simulink model "GOcontroll_Linux"  (R2018b)
settings: Solver=FixedStepDiscrete  StartTime=0.0  StopTime=5  FixedStep=0.01  RelTol=1e-3
PreLoadFcn:
  | librarySetup
PostLoadFcn:
  | core_info = evalc('feature(''numcores'')');
  | core_info_split = split(core_info, " ");
  | num_cores = core_info_split{12};
  | set_param(bdroot, "MakeCommand", ['make_rtw -j' num_cores]);
  | clear num_cores core_info core_info_split
libraries: GOcontroll_Moduline_Target x35, GOcontroll_Modbus x21, simulink x13, hdlsllib x8
settings Model: Creator=la_obwlf  LastModifiedBy=maud
settings DataIOCC: LimitDataPoints=on  SaveFormat=Array
settings OptimizationCC: BlockReduction=off  DefaultParameterBehavior=Inlined  LifeSpan=1
settings DebuggingCC: SolverPrmCheckMsg=warning  MultiTaskRateTransMsg=warning  ParameterPrecisionLossMsg=none  UnconnectedLineMsg=none  SFUnusedDataAndEventsDiag=none  SFUnexpectedBacktrackingDiag=warning  SFNoUnconditionalDefaultTransitionDiag=warning  SFUndirectedBroadcastEventsDiag=none  SFExecutionAtInitializationDiag=none  RCSCRenamedMsg=none  RCSCObservableMsg=none
settings HardwareCC: ProdBitPerLong=64  ProdLargestAtomicInteger=Long  ProdLargestAtomicFloat=Double  ProdLongLongMode=on  ProdHWDeviceType=ARM Compatible->ARM 64-bit (LP64)
settings ModelReferenceCC: PropagateSignalLabelsOutOfModel=off
settings SFSimCC: SimUseLocalCustomCode=off  MATLABDynamicMemAlloc=off
settings RTWCC: SystemTargetFile=ert_linux.tlc  MakeCommand=make_rtw -j24  TemplateMakefile=ert_linux_target_64.tmf  Description=Linux Embedded Coder  RTWUseLocalCustomCode=off
settings CodeAppCC: IgnoreCustomStorageClasses=off  StateflowObjectComments=on
settings STFCustomTargetCC: CombineOutputUpdateFcns=on  ERTCustomFileBanners=on  SupportContinuousTime=off  SupportNonInlinedSFcns=off  RemoveResetFunc=on  MATLABClassNameForMDSCustomization=Simulink.SoftwareTarget.ERTCustomization  SystemTargetFile=ert_linux.tlc
settings ERTTargetCC: MultiwordLength=2048  ParMdlRefBuildCompliant=off  CompOptLevelCompliant=off  ConcurrentExecutionCompliant=off  ModelStepFunctionPrototypeControlCompliant=off  CPPClassGenCompliant=off  UseToolchainInfoCompliant=off  GenerateASAP2=on  ERTCustomFileTemplate=ert_linux_file_process.tlc  PreserveExpressionOrder=on  ConvertIfToSwitch=off  SuppressUnreachableDefaultCases=off
settings ConfigComp: CovMetricSettings=dw  CovHtmlReporting=on  CovSaveCumulativeToWorkspaceVar=on  CovSaveSingleToWorkspaceVar=on  CovExternalEMLEnable=off  CovSFcnEnable=off

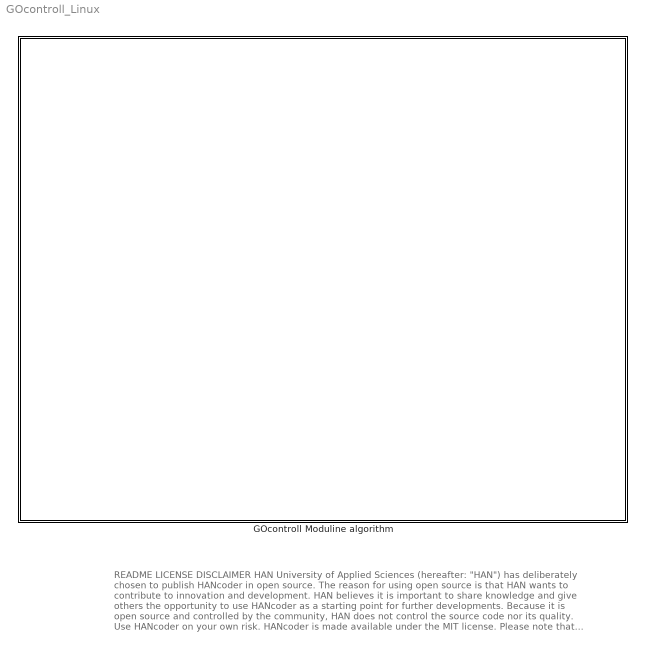
== system GOcontroll_Linux ==
  note: README
      |
      | LICENSE
      |
      | DISCLAIMER
      |
      | HAN University of Applied Sciences (hereafter: "HAN") has deliberately chosen
      | to publish HANcoder in open source. The reason for using open source is that
      | HAN wants to contribute to innovation and development. HAN believes it is
      | important to share knowledge and give others the opportunity to use HANcoder
      | as a starting point for further developments. Because it is open source and
      | controlled by the community, HAN does not control the source code nor its
      | quality. Use HANcoder on your own risk. HANcoder is made available under the
      | MIT license. Please note that this license contains an exclusion of liability.
  GOcontroll Moduline algorithm : Subsystem  mask(TopLevelSubsystem){}
      mask Display: image(imread('GOcontroll.png'))

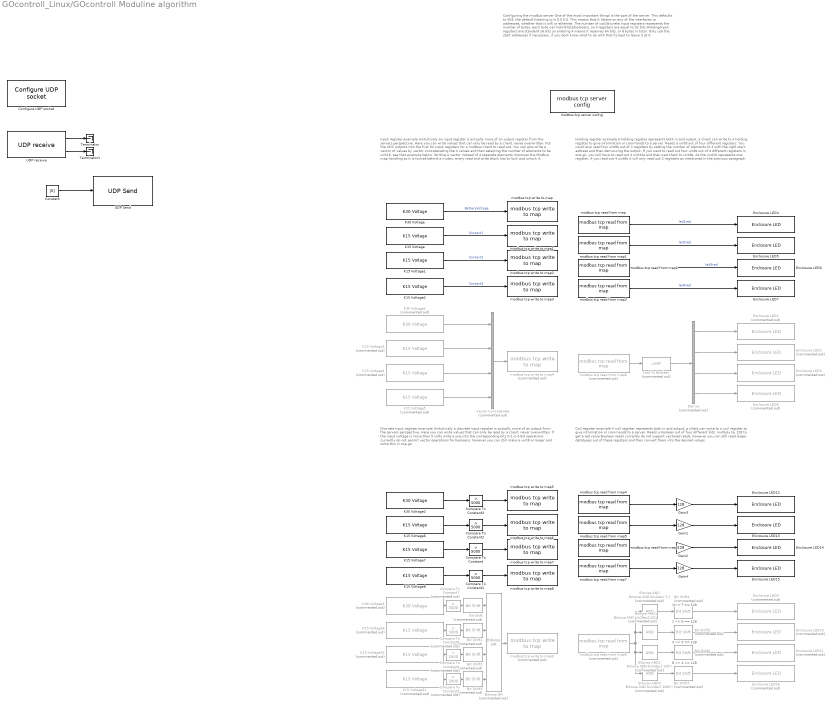
== system GOcontroll_Linux/GOcontroll Moduline algorithm ==
  note: 1 << 7 == 128
  note: Configuring the modbus server
      | One of the most important things is the port of the server.
      | This defaults to 503, the default listening ip is 0.0.0.0.
      | This means that it listens on any of the interfaces ip addresses,
      | whether that is wifi or ethernet.
      |
      | The number of coil/discrete input registers represents the number of bytes,
      | each byte can hold 8 bits/booleans, so 4 registers are equal to 32 bits
      |
      | Holding/input registers are standard 16 bits so entering 4 means it reserves
      | 64 bits, or 8 bytes in total.
      |
      | Only use the start addresses if necessary, if you dont know what to do with that
      | its best to leave it at 0
  note: Holding register example
      | A holding register represents both in and output, a client can write
      | to a holding register to give information or commands to a server.
      |
      | Reads a uint8 out of four different registers.
      | You could also read four uint8s out of 2 registers by setting
      | the number of elements to 4 with the right start address and then
      | demuxxing the output.
      |
      | If you want to read out four uin8s out of 4 different registers in one go, you will have to read out 4 uint16s
      | and then cast them to uint8s. As the uint16 represents one register, if you read out 4 uint8s it will only read out 2
      | registers as mentioned in the previous paragraph
  note: Input register example
      | Unituitively an input register is actually more of an output register from the servers perspective.
      | Here you can write values that can only be read by a client, never overwritten.
      |
      | Put the ADC outputs into the first for input registers for a modbus client to read out.
      |
      | You can also write a vector of values by vector concatenating the 4 values and then selecting
      | the number of elements to be uint16, see that example below.
      | Writing a vector instead of 4 seperate elements improves the Modbus map handling as it is
      | locked behind a mutex, every read and write block has to lock and unlock it.
  note: Coil register example
      | A coil register represents both in and output, a client can write
      | to a coil register to give information or commands to a server.
      |
      | Reads a boolean out of four different bits, multiply by 128 to get a led value
      |
      | Boolean reads currently do not support vectored reads, however you can still read larger datatypes out of these
      | registers and then convert them into the desired values.
  note: Discrete input register example
      | Unituitively a discrete input register is actually more of an output from the servers perspective.
      | Here you can write values that can only be read by a client, never overwritten.
      |
      | If the input voltage is more than 5 volts write a one into the corresponding bits 0-1-2-3
      |
      | Bit operations currently do not permit vector operations for booleans, however you can still
      | make a uint8 or larger and write this in one go.
  note: 2 << 6 == 128
  note: 4 << 5 == 128
  note: 8 << 4 == 128
  Bit Shift : hdlsllib/Logic and Bit Operations/Bit Shift  Commented=on  mode=Shift Left Logical  N=0
      settings: SourceProductName=HDL Coder  SourceProductBaseCode=HD
  Bit Shift1 : hdlsllib/Logic and Bit Operations/Bit Shift  Commented=on  mode=Shift Left Logical  N=1
      settings: SourceProductName=HDL Coder  SourceProductBaseCode=HD
  Bit Shift2 : hdlsllib/Logic and Bit Operations/Bit Shift  Commented=on  mode=Shift Left Logical  N=2
      settings: SourceProductName=HDL Coder  SourceProductBaseCode=HD
  Bit Shift3 : hdlsllib/Logic and Bit Operations/Bit Shift  Commented=on  mode=Shift Left Logical  N=3
      settings: SourceProductName=HDL Coder  SourceProductBaseCode=HD
  Bit Shift4 : hdlsllib/Logic and Bit Operations/Bit Shift  Commented=on  mode=Shift Left Logical  N=7
      settings: SourceProductName=HDL Coder  SourceProductBaseCode=HD
  Bit Shift5 : hdlsllib/Logic and Bit Operations/Bit Shift  Commented=on  mode=Shift Left Logical  N=6
      settings: SourceProductName=HDL Coder  SourceProductBaseCode=HD
  Bit Shift6 : hdlsllib/Logic and Bit Operations/Bit Shift  Commented=on  mode=Shift Left Logical  N=5
      settings: SourceProductName=HDL Coder  SourceProductBaseCode=HD
  Bit Shift7 : hdlsllib/Logic and Bit Operations/Bit Shift  Commented=on  mode=Shift Left Logical  N=4
      settings: SourceProductName=HDL Coder  SourceProductBaseCode=HD
  Bitwise AND : simulink/Logic and Bit Operations/Bitwise Operator  Commented=on  logicop=AND  UseBitMask=on  BitMask=bin2dec('1')  BitMaskRealWorld=Stored Integer
  Bitwise AND1 : simulink/Logic and Bit Operations/Bitwise Operator  Commented=on  logicop=AND  UseBitMask=on  BitMask=bin2dec('10')  BitMaskRealWorld=Stored Integer
  Bitwise AND2 : simulink/Logic and Bit Operations/Bitwise Operator  Commented=on  logicop=AND  UseBitMask=on  BitMask=bin2dec('100')  BitMaskRealWorld=Stored Integer
  Bitwise AND3 : simulink/Logic and Bit Operations/Bitwise Operator  Commented=on  logicop=AND  UseBitMask=on  BitMask=bin2dec('1000')  BitMaskRealWorld=Stored Integer
  Bitwise OR : simulink/Logic and Bit Operations/Bitwise Operator  Commented=on  logicop=OR  UseBitMask=off  NumInputPorts=4  BitMask=bin2dec('11011001')  BitMaskRealWorld=Stored Integer
  Cast To Boolean : DataTypeConversion  Commented=on  OutDataTypeStr=uint8
  Compare To Constant{,1..3} (4 alike) : simulink/Logic and Bit Operations/Compare To Constant  relop=>  const=5000  OutDataTypeStr=boolean
  Compare To Constant{4..7} (4 alike) : simulink/Logic and Bit Operations/Compare To Constant  Commented=on  relop=>  const=5000  OutDataTypeStr=uint8
  Configure UDP socket : GOcontroll_Moduline_Target/Network/UDP/Configure UDP socket  port=9001  ip='0.0.0.0'  broadcast=on  tsamp=0.01
      settings: SourceProductName=GOcontroll Moduline
  Constant : Constant  Value=[0]  OutDataTypeStr=uint8
  Demux : Demux  Commented=on
  Enclosure LED1 : GOcontroll_Moduline_Target/Enclosure LED's/Enclosure LED  Tag=HANcoder_GOcontroll_Moduline_IV  Commented=on  led=1  color=Red
      settings: SourceProductName=GOcontroll Moduline
  Enclosure LED10 : GOcontroll_Moduline_Target/Enclosure LED's/Enclosure LED  Tag=HANcoder_GOcontroll_Moduline_IV  Commented=on  led=2  color=Red
      settings: SourceProductName=GOcontroll Moduline
  Enclosure LED11 : GOcontroll_Moduline_Target/Enclosure LED's/Enclosure LED  Tag=HANcoder_GOcontroll_Moduline_IV  Commented=on  led=3  color=Red
      settings: SourceProductName=GOcontroll Moduline
  Enclosure LED12 : GOcontroll_Moduline_Target/Enclosure LED's/Enclosure LED  Tag=HANcoder_GOcontroll_Moduline_IV  led=1  color=Green
      settings: SourceProductName=GOcontroll Moduline
  Enclosure LED13 : GOcontroll_Moduline_Target/Enclosure LED's/Enclosure LED  Tag=HANcoder_GOcontroll_Moduline_IV  led=2  color=Green
      settings: SourceProductName=GOcontroll Moduline
  Enclosure LED14 : GOcontroll_Moduline_Target/Enclosure LED's/Enclosure LED  Tag=HANcoder_GOcontroll_Moduline_IV  led=3  color=Green
      settings: SourceProductName=GOcontroll Moduline
  Enclosure LED15 : GOcontroll_Moduline_Target/Enclosure LED's/Enclosure LED  Tag=HANcoder_GOcontroll_Moduline_IV  led=4  color=Green
      settings: SourceProductName=GOcontroll Moduline
  Enclosure LED16 : GOcontroll_Moduline_Target/Enclosure LED's/Enclosure LED  Tag=HANcoder_GOcontroll_Moduline_IV  Commented=on  led=4  color=Red
      settings: SourceProductName=GOcontroll Moduline
  Enclosure LED2 : GOcontroll_Moduline_Target/Enclosure LED's/Enclosure LED  Tag=HANcoder_GOcontroll_Moduline_IV  Commented=on  led=2  color=Red
      settings: SourceProductName=GOcontroll Moduline
  Enclosure LED3 : GOcontroll_Moduline_Target/Enclosure LED's/Enclosure LED  Tag=HANcoder_GOcontroll_Moduline_IV  Commented=on  led=3  color=Red
      settings: SourceProductName=GOcontroll Moduline
  Enclosure LED4 : GOcontroll_Moduline_Target/Enclosure LED's/Enclosure LED  Tag=HANcoder_GOcontroll_Moduline_IV  led=1  color=Red
      settings: SourceProductName=GOcontroll Moduline
  Enclosure LED5 : GOcontroll_Moduline_Target/Enclosure LED's/Enclosure LED  Tag=HANcoder_GOcontroll_Moduline_IV  led=2  color=Red
      settings: SourceProductName=GOcontroll Moduline
  Enclosure LED6 : GOcontroll_Moduline_Target/Enclosure LED's/Enclosure LED  Tag=HANcoder_GOcontroll_Moduline_IV  led=3  color=Red
      settings: SourceProductName=GOcontroll Moduline
  Enclosure LED7 : GOcontroll_Moduline_Target/Enclosure LED's/Enclosure LED  Tag=HANcoder_GOcontroll_Moduline_IV  led=4  color=Red
      settings: SourceProductName=GOcontroll Moduline
  Enclosure LED8 : GOcontroll_Moduline_Target/Enclosure LED's/Enclosure LED  Tag=HANcoder_GOcontroll_Moduline_IV  Commented=on  led=4  color=Red
      settings: SourceProductName=GOcontroll Moduline
  Enclosure LED9 : GOcontroll_Moduline_Target/Enclosure LED's/Enclosure LED  Tag=HANcoder_GOcontroll_Moduline_IV  Commented=on  led=1  color=Red
      settings: SourceProductName=GOcontroll Moduline
  Gain{1..4} (4 alike) : Gain  Gain=128  ParamDataTypeStr=uint8  OutDataTypeStr=uint8
  K15 Voltage : GOcontroll_Moduline_Target/Supply control/K15 Voltage  Tag=HANcoder_GOcontroll_Moduline_IV  tsamp=0.1  k15pin=K15-1 (Connector C pin 2)
      settings: SourceProductName=GOcontroll Moduline
  K15 Voltage1 : GOcontroll_Moduline_Target/Supply control/K15 Voltage  Tag=HANcoder_GOcontroll_Moduline_IV  tsamp=0.1  k15pin=K15-2 (Connector C pin 3)
      settings: SourceProductName=GOcontroll Moduline
  K15 Voltage10 : GOcontroll_Moduline_Target/Supply control/K15 Voltage  Tag=HANcoder_GOcontroll_Moduline_IV  Commented=on  tsamp=0.1  k15pin=K15-2 (Connector C pin 3)
      settings: SourceProductName=GOcontroll Moduline
  K15 Voltage11 : GOcontroll_Moduline_Target/Supply control/K15 Voltage  Tag=HANcoder_GOcontroll_Moduline_IV  Commented=on  tsamp=0.1  k15pin=K15-3 (Connector C pin 4)
      settings: SourceProductName=GOcontroll Moduline
  K15 Voltage2 : GOcontroll_Moduline_Target/Supply control/K15 Voltage  Tag=HANcoder_GOcontroll_Moduline_IV  tsamp=0.1  k15pin=K15-3 (Connector C pin 4)
      settings: SourceProductName=GOcontroll Moduline
  K15 Voltage3 : GOcontroll_Moduline_Target/Supply control/K15 Voltage  Tag=HANcoder_GOcontroll_Moduline_IV  Commented=on  tsamp=0.1  k15pin=K15-1 (Connector C pin 2)
      settings: SourceProductName=GOcontroll Moduline
  K15 Voltage4 : GOcontroll_Moduline_Target/Supply control/K15 Voltage  Tag=HANcoder_GOcontroll_Moduline_IV  Commented=on  tsamp=0.1  k15pin=K15-2 (Connector C pin 3)
      settings: SourceProductName=GOcontroll Moduline
  K15 Voltage5 : GOcontroll_Moduline_Target/Supply control/K15 Voltage  Tag=HANcoder_GOcontroll_Moduline_IV  Commented=on  tsamp=0.1  k15pin=K15-3 (Connector C pin 4)
      settings: SourceProductName=GOcontroll Moduline
  K15 Voltage6 : GOcontroll_Moduline_Target/Supply control/K15 Voltage  Tag=HANcoder_GOcontroll_Moduline_IV  tsamp=0.1  k15pin=K15-1 (Connector C pin 2)
      settings: SourceProductName=GOcontroll Moduline
  K15 Voltage7 : GOcontroll_Moduline_Target/Supply control/K15 Voltage  Tag=HANcoder_GOcontroll_Moduline_IV  tsamp=0.1  k15pin=K15-2 (Connector C pin 3)
      settings: SourceProductName=GOcontroll Moduline
  K15 Voltage8 : GOcontroll_Moduline_Target/Supply control/K15 Voltage  Tag=HANcoder_GOcontroll_Moduline_IV  tsamp=0.1  k15pin=K15-3 (Connector C pin 4)
      settings: SourceProductName=GOcontroll Moduline
  K15 Voltage9 : GOcontroll_Moduline_Target/Supply control/K15 Voltage  Tag=HANcoder_GOcontroll_Moduline_IV  Commented=on  tsamp=0.1  k15pin=K15-1 (Connector C pin 2)
      settings: SourceProductName=GOcontroll Moduline
  K30 Voltage : GOcontroll_Moduline_Target/Supply control/K30 Voltage  Tag=HANcoder_GOcontroll_Moduline_IV  tsamp=0.1
      settings: SourceProductName=GOcontroll Moduline
  K30 Voltage1 : GOcontroll_Moduline_Target/Supply control/K30 Voltage  Tag=HANcoder_GOcontroll_Moduline_IV  Commented=on  tsamp=0.1
      settings: SourceProductName=GOcontroll Moduline
  K30 Voltage2 : GOcontroll_Moduline_Target/Supply control/K30 Voltage  Tag=HANcoder_GOcontroll_Moduline_IV  tsamp=0.1
      settings: SourceProductName=GOcontroll Moduline
  K30 Voltage3 : GOcontroll_Moduline_Target/Supply control/K30 Voltage  Tag=HANcoder_GOcontroll_Moduline_IV  Commented=on  tsamp=0.1
      settings: SourceProductName=GOcontroll Moduline
  Terminator : Terminator
  Terminator1 : Terminator
  UDP Send : GOcontroll_Moduline_Target/Network/UDP/UDP Send  input_type=off  id=0  ip='0.0.0.0'  port=0  tsamp=1
      settings: SourceProductName=GOcontroll Moduline
  UDP receive : GOcontroll_Moduline_Target/Network/UDP/UDP receive  input_type=off  id=0  buff_len=1  tsamp=1
      settings: SourceProductName=GOcontroll Moduline
  Vector Concatenate : Concatenate  Commented=on  NumInputs=4
  modbus tcp read from map : GOcontroll_Modbus/TCP/modbus tcp read from map  block_type=Holding register  data_type=uint8  address=0  length=1  bit=0  tsamp=0.1
      settings: SourceProductName=GOcontroll Modbus
  modbus tcp read from map1 : GOcontroll_Modbus/TCP/modbus tcp read from map  block_type=Holding register  data_type=uint8  address=1  length=1  bit=0  tsamp=0.1
      settings: SourceProductName=GOcontroll Modbus
  modbus tcp read from map2 : GOcontroll_Modbus/TCP/modbus tcp read from map  block_type=Holding register  data_type=uint8  address=2  length=1  bit=0  tsamp=0.1
      settings: SourceProductName=GOcontroll Modbus
  modbus tcp read from map3 : GOcontroll_Modbus/TCP/modbus tcp read from map  block_type=Holding register  data_type=uint8  address=3  length=1  bit=0  tsamp=0.1
      settings: SourceProductName=GOcontroll Modbus
  modbus tcp read from map4 : GOcontroll_Modbus/TCP/modbus tcp read from map  block_type=Coil  data_type=boolean  address=0  length=1  bit=0  tsamp=0.1
      settings: SourceProductName=GOcontroll Modbus
  modbus tcp read from map5 : GOcontroll_Modbus/TCP/modbus tcp read from map  block_type=Coil  data_type=boolean  address=0  length=1  bit=1  tsamp=0.1
      settings: SourceProductName=GOcontroll Modbus
  modbus tcp read from map6 : GOcontroll_Modbus/TCP/modbus tcp read from map  block_type=Coil  data_type=boolean  address=0  length=1  bit=2  tsamp=0.1
      settings: SourceProductName=GOcontroll Modbus
  modbus tcp read from map7 : GOcontroll_Modbus/TCP/modbus tcp read from map  block_type=Coil  data_type=boolean  address=0  length=1  bit=3  tsamp=0.1
      settings: SourceProductName=GOcontroll Modbus
  modbus tcp read from map8 : GOcontroll_Modbus/TCP/modbus tcp read from map  Commented=on  block_type=Holding register  data_type=uint16  address=0  length=4  bit=0  tsamp=0.1
      settings: SourceProductName=GOcontroll Modbus
  modbus tcp read from map9 : GOcontroll_Modbus/TCP/modbus tcp read from map  Commented=on  block_type=Coil  data_type=uint8  address=0  length=1  bit=0  tsamp=0.1
      settings: SourceProductName=GOcontroll Modbus
  modbus tcp server config : GOcontroll_Modbus/TCP/modbus tcp server config  ip="\"0.0.0.0\""  port=503  coils_addr=0  coils_num=1  discrete_in_addr=0  discrete_in_num=1  holding_addr=0  holding_num=4  input_addr=0  input_num=4
      settings: SourceProductName=GOcontroll Modbus
  modbus tcp write to map : GOcontroll_Modbus/TCP/modbus tcp write to map  block_type=Input register  data_type=uint16  address=0  length=1  bit=0  tsamp=0.1
      settings: SourceProductName=GOcontroll Modbus
  modbus tcp write to map1 : GOcontroll_Modbus/TCP/modbus tcp write to map  block_type=Input register  data_type=uint16  address=1  length=1  bit=0  tsamp=0.1
      settings: SourceProductName=GOcontroll Modbus
  modbus tcp write to map2 : GOcontroll_Modbus/TCP/modbus tcp write to map  block_type=Input register  data_type=uint16  address=2  length=1  bit=0  tsamp=0.1
      settings: SourceProductName=GOcontroll Modbus
  modbus tcp write to map3 : GOcontroll_Modbus/TCP/modbus tcp write to map  block_type=Input register  data_type=uint16  address=3  length=1  bit=0  tsamp=0.1
      settings: SourceProductName=GOcontroll Modbus
  modbus tcp write to map4 : GOcontroll_Modbus/TCP/modbus tcp write to map  Commented=on  block_type=Input register  data_type=uint16  address=0  length=4  bit=0  tsamp=0.1
      settings: SourceProductName=GOcontroll Modbus
  modbus tcp write to map5 : GOcontroll_Modbus/TCP/modbus tcp write to map  block_type=Discrete input  data_type=boolean  address=0  length=1  bit=0  tsamp=0.1
      settings: SourceProductName=GOcontroll Modbus
  modbus tcp write to map6 : GOcontroll_Modbus/TCP/modbus tcp write to map  block_type=Discrete input  data_type=boolean  address=0  length=1  bit=1  tsamp=0.1
      settings: SourceProductName=GOcontroll Modbus
  modbus tcp write to map7 : GOcontroll_Modbus/TCP/modbus tcp write to map  block_type=Discrete input  data_type=boolean  address=0  length=1  bit=3  tsamp=0.1
      settings: SourceProductName=GOcontroll Modbus
  modbus tcp write to map8 : GOcontroll_Modbus/TCP/modbus tcp write to map  block_type=Discrete input  data_type=boolean  address=0  length=1  bit=3  tsamp=0.1
      settings: SourceProductName=GOcontroll Modbus
  modbus tcp write to map9 : GOcontroll_Modbus/TCP/modbus tcp write to map  Commented=on  block_type=Discrete input  data_type=uint8  address=0  length=1  bit=0  tsamp=0.1
      settings: SourceProductName=GOcontroll Modbus
  wires:
  K15 Voltage/1 -> modbus tcp write to map1/1  "Contact1"
  K15 Voltage2/1 -> modbus tcp write to map3/1  "Contact3"
  K30 Voltage/1 -> modbus tcp write to map/1  "BatteryVoltage"
  K15 Voltage1/1 -> modbus tcp write to map2/1  "Contact2"
  modbus tcp read from map/1 -> Enclosure LED4/1  "led1red"
  modbus tcp read from map1/1 -> Enclosure LED5/1  "led2red"
  modbus tcp read from map2/1 -> Enclosure LED6/1  "led3red"
  modbus tcp read from map3/1 -> Enclosure LED7/1  "led4red"
  K15 Voltage4/1 -> Vector Concatenate/3
  K30 Voltage1/1 -> Vector Concatenate/1
  K15 Voltage5/1 -> Vector Concatenate/4
  K15 Voltage3/1 -> Vector Concatenate/2
  Vector Concatenate/1 -> modbus tcp write to map4/1
  Demux/4 -> Enclosure LED8/1
  Demux/3 -> Enclosure LED3/1
  Demux/2 -> Enclosure LED2/1
  Demux/1 -> Enclosure LED1/1
  modbus tcp read from map8/1 -> Cast To Boolean/1
  Cast To Boolean/1 -> Demux/1
  modbus tcp read from map9/1 -> Bitwise AND1/1, Bitwise AND/1, Bitwise AND3/1, Bitwise AND2/1
  Bit Shift4/1 -> Enclosure LED9/1
  Bit Shift5/1 -> Enclosure LED10/1
  Bit Shift6/1 -> Enclosure LED11/1
  Bit Shift7/1 -> Enclosure LED16/1
  modbus tcp read from map7/1 -> Gain4/1
  modbus tcp read from map6/1 -> Gain2/1
  modbus tcp read from map5/1 -> Gain1/1
  modbus tcp read from map4/1 -> Gain3/1
  K15 Voltage7/1 -> Compare To Constant/1
  Compare To Constant3/1 -> modbus tcp write to map5/1
  K15 Voltage8/1 -> Compare To Constant1/1
  Compare To Constant2/1 -> modbus tcp write to map6/1
  Compare To Constant1/1 -> modbus tcp write to map8/1
  Compare To Constant/1 -> modbus tcp write to map7/1
  K15 Voltage6/1 -> Compare To Constant2/1
  K30 Voltage2/1 -> Compare To Constant3/1
  K30 Voltage3/1 -> Compare To Constant7/1
  K15 Voltage9/1 -> Compare To Constant6/1
  K15 Voltage11/1 -> Compare To Constant5/1
  K15 Voltage10/1 -> Compare To Constant4/1
  Compare To Constant7/1 -> Bit Shift/1
  Compare To Constant5/1 -> Bit Shift3/1
  Compare To Constant4/1 -> Bit Shift2/1
  Compare To Constant6/1 -> Bit Shift1/1
  Bit Shift/1 -> Bitwise OR/1
  Bit Shift1/1 -> Bitwise OR/2
  Bit Shift2/1 -> Bitwise OR/3
  Bit Shift3/1 -> Bitwise OR/4
  Bitwise OR/1 -> modbus tcp write to map9/1
  Gain4/1 -> Enclosure LED15/1
  Gain2/1 -> Enclosure LED14/1
  Gain1/1 -> Enclosure LED13/1
  Gain3/1 -> Enclosure LED12/1
  Bitwise AND/1 -> Bit Shift4/1
  Bitwise AND1/1 -> Bit Shift5/1
  Bitwise AND2/1 -> Bit Shift6/1
  Bitwise AND3/1 -> Bit Shift7/1
  UDP receive/2 -> Terminator1/1
  UDP receive/1 -> Terminator/1
  Constant/1 -> UDP Send/1
